simulink model "SimulinkPID_lift"  (R2021a)
settings: Solver=VariableStepAuto  StartTime=0.0  StopTime=10.0  RelTol=1e-3
settings Model: Creator=ACER  LastModifiedBy=ACER

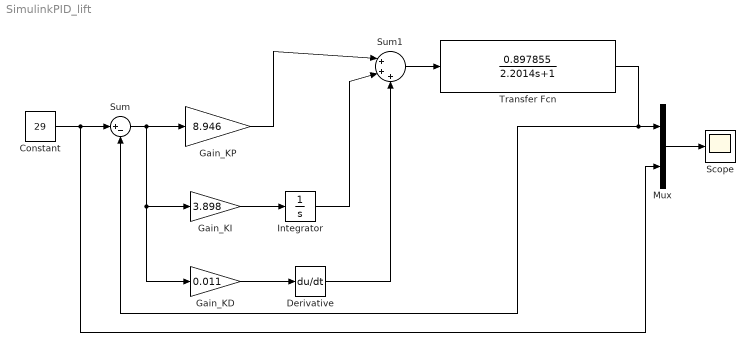
== system SimulinkPID_lift ==
  Constant : Constant  Value=29
  Derivative : Derivative
  Gain_KD : Gain  Gain=0.011
  Gain_KI : Gain  Gain=3.898
  Gain_KP : Gain  Gain=8.946
  Integrator : Integrator
  Mux : Mux  Inputs=2
  Scope : Scope
  Sum : Sum  Inputs=|+-
  Sum1 : Sum  Inputs=|+++
  Transfer Fcn : TransferFcn  Numerator=[0.897855]  Denominator=[2.2014 1]
  wires:
  Constant/1 -> Mux/2, Sum/1
  Gain_KI/1 -> Integrator/1
  Gain_KD/1 -> Derivative/1
  Gain_KP/1 -> Sum1/1
  Integrator/1 -> Sum1/2
  Derivative/1 -> Sum1/3
  Sum1/1 -> Transfer Fcn/1
  Transfer Fcn/1 -> Mux/1, Sum/2
  Sum/1 -> Gain_KD/1, Gain_KI/1, Gain_KP/1
  Mux/1 -> Scope/1
